simulink model "Example_6"  (R2020b)
settings: Solver=VariableStepAuto  StartTime=0.0  StopTime=0.1  RelTol=1e-3
libraries: fl_lib x8, nesl_utility x4, dspsigops x3, ee_lib x2
settings Model: Creator=zaliyazici  LastModifiedBy=zaliyazici

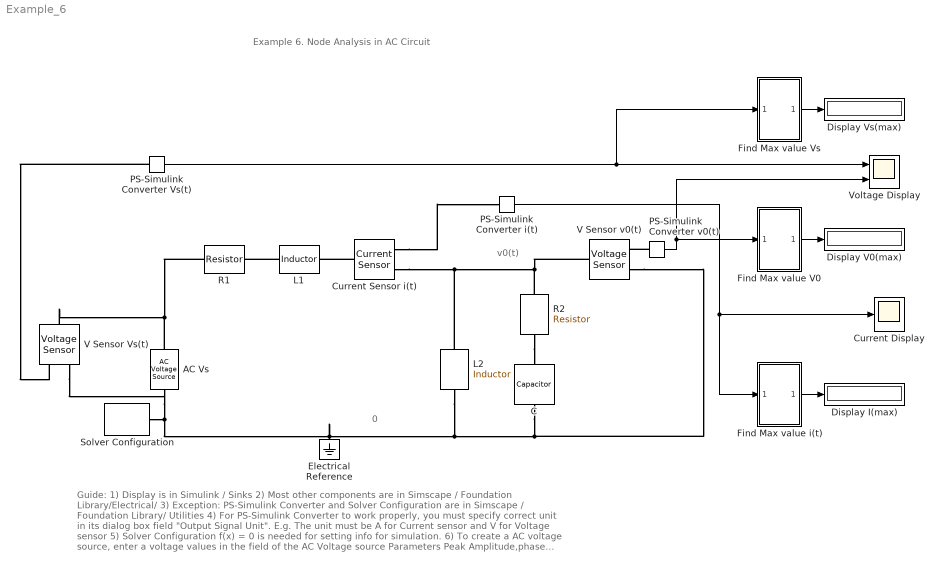
== system Example_6 ==
  note: Guide:
      | 1) Display is in Simulink / Sinks
      | 2) Most other components are in Simscape / Foundation Library/Electrical/
      | 3) Exception: PS-Simulink Converter and Solver Configuration are in Simscape / Foundation Library/ Utilities
      | 4) For PS-Simulink Converter to work properly, you must specify correct unit in its dialog box field "Output Signal Unit".
      | E.g. The unit must be A for Current sensor and V for Voltage sensor
      | 5) Solver Configuration f(x) = 0 is needed for setting info for simulation.
      | 6) To create a AC voltage source, enter a voltage values in the field of the AC Voltage source Parameters Peak Amplitude,phase shift and Frequency. Use 90 degree in phase o conver cosine signal.
      | 7) To create "Annotation", double-click a location on project page and select "Create annotation" from the prompt. Then, type any text you want to clarify your circuit. E.g. "Display for Current".
      | 8) To understand how to use a component, right-click on the component and select "Help".
      | Measurement: $v_s(t), v_0(t)$ , and current $i(t)$
  note: Example 6. Node Analysis in AC Circuit
  note: 0
  note: v0(t)
  AC Vs : fl_lib/Electrical/Electrical Sources/AC Voltage Source  amp=36 V  shift=90 deg  frequency=60 Hz  omega=0 rad/s
      settings: AttributesFormatString=|
      | %<amp> %<amp_unit>
      | %<frequency> %<frequency_unit>
      | %<shift> %<shift_unit>
  C : fl_lib/Electrical/Electrical Elements/Capacitor  c=100 uF  r=1e-6 Ohm  g=0 1/Ohm  i_specify=off  i_priority=None  i=0 A  i_nominal_specify=off  i_nominal_unit=A  i_nominal_value=1  v_specify=off  v_priority=None  v=0 V  v_nominal_specify=off  v_nominal_unit=V  v_nominal_value=1  vc_specify=on  vc_priority=High  vc=0 V  vc_nominal_specify=off  vc_nominal_unit=V  vc_nominal_value=1
      settings: AttributesFormatString=%<c> %<c_unit>
  Current Display : Scope
  Current Sensor i(t) : fl_lib/Electrical/Electrical Sensors/Current Sensor
  Display I(max) : Display
  Display V0(max) : Display
  Display Vs(max) : Display
  Electrical Reference : fl_lib/Electrical/Electrical Elements/Electrical Reference
  Find Max value V0 : Subsystem
  Find Max value Vs : Subsystem
  Find Max value i(t) : Subsystem
  L1 : fl_lib/Electrical/Electrical Elements/Inductor  l=50 mH  r=0 Ohm  g=1e-9 1/Ohm  i_specify=off  i_priority=None  i=0 A  i_nominal_specify=off  i_nominal_unit=A  i_nominal_value=1  v_specify=off  v_priority=None  v=0 V  v_nominal_specify=off  v_nominal_unit=V  v_nominal_value=1  i_L_specify=on  i_L_priority=High  i_L=0 mA  i_L_nominal_specify=off  i_L_nominal_unit=A  i_L_nominal_value=1
      settings: AttributesFormatString=%<l> %<l_unit>
  L2 : fl_lib/Electrical/Electrical Elements/Inductor  l=100 mH  r=0 Ohm  g=1e-9 1/Ohm  i_specify=off  i_priority=None  i=0 A  i_nominal_specify=off  i_nominal_unit=A  i_nominal_value=1  v_specify=off  v_priority=None  v=0 V  v_nominal_specify=off  v_nominal_unit=V  v_nominal_value=1  i_L_specify=on  i_L_priority=High  i_L=0 mA  i_L_nominal_specify=off  i_L_nominal_unit=A  i_L_nominal_value=1
      settings: AttributesFormatString=%<l> %<l_unit>
  PS-Simulink Converter Vs(t) : nesl_utility/PS-Simulink Converter  PhysicalDomain=network_engine_domain  SubClassName=ps_output  LeftPortType=input  RightPortType=output  PseudoPeriodic=off  Frequencies=[]  Unit=V  AffineConversion=off
  PS-Simulink Converter i(t) : nesl_utility/PS-Simulink Converter  PhysicalDomain=network_engine_domain  SubClassName=ps_output  LeftPortType=input  RightPortType=output  PseudoPeriodic=off  Frequencies=[]  Unit=A  AffineConversion=off
  PS-Simulink Converter v0(t) : nesl_utility/PS-Simulink Converter  PhysicalDomain=network_engine_domain  SubClassName=ps_output  LeftPortType=input  RightPortType=output  PseudoPeriodic=off  Frequencies=[]  Unit=V  AffineConversion=off
  R1 : ee_lib/Passive/Resistor  R=100 Ohm  R_tol=5  enable_R_tol=0  tol_distribution=1  nSigma=4  enable_operating_limits=0  operating_limit_action=2  max_working_voltage=100 V  power_rating=1 W  enable_faults=0  fault_action=1  R_faulted=inf Ohm  enable_temporal_fault=0  t_fault=1 s  enable_behavioral_fault=0  max_permissible_current=1 A  t_fail_on_current=1 s  noise_mode=0  sample_time=1e-3 s  repeatability=1  auto_seed=57050912  user_seed=0  Tdevice=25 degC  alpha=3.93e-3 1/K  Tmeas=25 degC  thermal_mass=100 J/K  power_derating_T1=70 degC  power_derating_T2=155 degC  operating_temperature_range_vec=[-50, 150] degC  temperature_specify=off  temperature_priority=High  temperature=298.15 K  temperature_nominal_specify=off  temperature_nominal_unit=K  temperature_nominal_value=1
      settings: AttributesFormatString=%<R> %<R_unit>
  R2 : ee_lib/Passive/Resistor  R=80 Ohm  R_tol=5  enable_R_tol=0  tol_distribution=1  nSigma=4  enable_operating_limits=0  operating_limit_action=2  max_working_voltage=100 V  power_rating=1 W  enable_faults=0  fault_action=1  R_faulted=inf Ohm  enable_temporal_fault=0  t_fault=1 s  enable_behavioral_fault=0  max_permissible_current=1 A  t_fail_on_current=1 s  noise_mode=0  sample_time=1e-3 s  repeatability=1  auto_seed=1493414552  user_seed=0  Tdevice=25 degC  alpha=3.93e-3 1/K  Tmeas=25 degC  thermal_mass=100 J/K  power_derating_T1=70 degC  power_derating_T2=155 degC  operating_temperature_range_vec=[-50, 150] degC  temperature_specify=off  temperature_priority=High  temperature=298.15 K  temperature_nominal_specify=off  temperature_nominal_unit=K  temperature_nominal_value=1
      settings: AttributesFormatString=%<R> %<R_unit>
  Solver Configuration : nesl_utility/Solver Configuration  PhysicalDomain=network_engine_domain  SubClassName=solver  LeftPortType=input  RightPortType=generic  Tones=[]  Harmonics=[]  SimulateNoise=off  Profile=off  UseLocalSampling=off  EnableSwitchedLinearOptims=on  FrequencyDomain=off  UseCCode=off  RelTol=0.001  AbsTol=1e-06  MinStep=1e-09  ToWorkspace=off  RevertToSquareIcSolve=off  NumHomotopyIterations=100  PhasorMode=off  PhasorModeNumHarmonics=1  DoDC=off  ResidualTolerance=1e-09  UseLocalSolver=off  LocalSolverChoice=NE_BACKWARD_EULER_ADVANCER  LocalSolverSampleTime=0.001  DoFixedCost=off  MaxNonlinIter=3  MaxModeIter=2  ComputeImpulses=off  ImpulseIterations=2  LinearAlgebra=auto  EquationFormulation=NE_TIME_EF  DelaysMemoryBudget=1024  AutomaticFiltering=on  FilteringTimeConstant=0.001  PartitionStorageMethod=AS_NEEDED  PartitionMemoryBudget=1024  PartitionMethod=ROBUST
  V Sensor Vs(t) : fl_lib/Electrical/Electrical Sensors/Voltage Sensor
  V Sensor v0(t) : fl_lib/Electrical/Electrical Sensors/Voltage Sensor
  Voltage Display : Scope  NumInputPorts=2
  wires:
  PS-Simulink Converter v0(t)/1 -> Find Max value V0/1(In1), Voltage Display/2
  PS-Simulink Converter Vs(t)/1 -> Voltage Display/1, Find Max value Vs/1(In1)
  Find Max value V0/1(Out2) -> Display V0(max)/1
  Find Max value i(t)/1(Out2) -> Display I(max)/1
  Find Max value Vs/1(Out2) -> Display Vs(max)/1
  PS-Simulink Converter i(t)/1 -> Find Max value i(t)/1(In1), Current Display/1
  connections:
  V Sensor Vs(t)/RConn2 -- AC Vs/RConn1 -- Solver Configuration/RConn1 -- L2/RConn1 -- C/RConn1 -- V Sensor v0(t)/RConn2 -- Electrical Reference/LConn1
  PS-Simulink Converter v0(t)/LConn1 -- V Sensor v0(t)/RConn1
  AC Vs/LConn1 -- R1/LConn1 -- V Sensor Vs(t)/LConn1
  PS-Simulink Converter Vs(t)/LConn1 -- V Sensor Vs(t)/RConn1
  L2/LConn1 -- Current Sensor i(t)/RConn2 -- R2/LConn1 -- V Sensor v0(t)/LConn1
  R2/RConn1 -- C/LConn1
  L1/LConn1 -- R1/RConn1
  Current Sensor i(t)/LConn1 -- L1/RConn1
  Current Sensor i(t)/RConn1 -- PS-Simulink Converter i(t)/LConn1

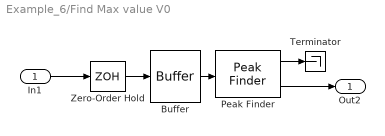
== system Example_6/Find Max value V0 ==
  In1 : Inport
  Buffer : Buffer  N=256  OutputFrames=off
  Peak Finder : dspsigops/Peak Finder  polarity=Maxima  outputIdx=off  outputVal=on  maxPeaks=1  NoiseDistinguish=off  thresh=0  roundingMode=Floor  overflowMode=off
      settings: SourceProductBaseCode=DS  allowOverrides=off
  Terminator : Terminator
  Zero-Order Hold : ZeroOrderHold  SampleTime=1e-4
  Out2 : Outport
  wires:
  Buffer/1 -> Peak Finder/1
  Zero-Order Hold/1 -> Buffer/1
  Peak Finder/2 -> Out2/1
  Peak Finder/1 -> Terminator/1
  In1/1 -> Zero-Order Hold/1

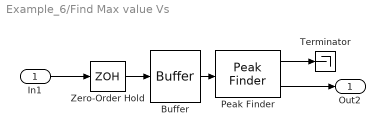
== system Example_6/Find Max value Vs ==
  In1 : Inport
  Buffer : Buffer  N=256  OutputFrames=off
  Peak Finder : dspsigops/Peak Finder  polarity=Maxima  outputIdx=off  outputVal=on  maxPeaks=1  NoiseDistinguish=off  thresh=0  roundingMode=Floor  overflowMode=off
      settings: SourceProductBaseCode=DS  allowOverrides=off
  Terminator : Terminator
  Zero-Order Hold : ZeroOrderHold  SampleTime=1e-4
  Out2 : Outport
  wires:
  Buffer/1 -> Peak Finder/1
  Zero-Order Hold/1 -> Buffer/1
  Peak Finder/2 -> Out2/1
  Peak Finder/1 -> Terminator/1
  In1/1 -> Zero-Order Hold/1

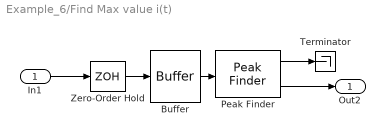
== system Example_6/Find Max value i(t) ==
  In1 : Inport
  Buffer : Buffer  N=256  OutputFrames=off
  Peak Finder : dspsigops/Peak Finder  polarity=Maxima  outputIdx=off  outputVal=on  maxPeaks=1  NoiseDistinguish=off  thresh=0  roundingMode=Floor  overflowMode=off
      settings: SourceProductBaseCode=DS  allowOverrides=off
  Terminator : Terminator
  Zero-Order Hold : ZeroOrderHold  SampleTime=1e-4
  Out2 : Outport
  wires:
  Buffer/1 -> Peak Finder/1
  Zero-Order Hold/1 -> Buffer/1
  Peak Finder/2 -> Out2/1
  Peak Finder/1 -> Terminator/1
  In1/1 -> Zero-Order Hold/1
